simulink model "EV_Regenerative_Braking_Test_FINAL"  (R2021a)
settings: Solver=VariableStepAuto  StartTime=0.0  StopTime=2  RelTol=1e-3
undefined symbols (not defined in the file): Ion, Lithium
libraries: spsBatteryLib x1, pid_lib x1, spsDCMachineLib x1, eePwmGenerator x1, spsTwoQuadrantDCDCConverterLib x1, spsVoltageMeasurementLib x1, spspowerguiLib x1
settings Model: Creator=Adrija  LastModifiedBy=Adrija

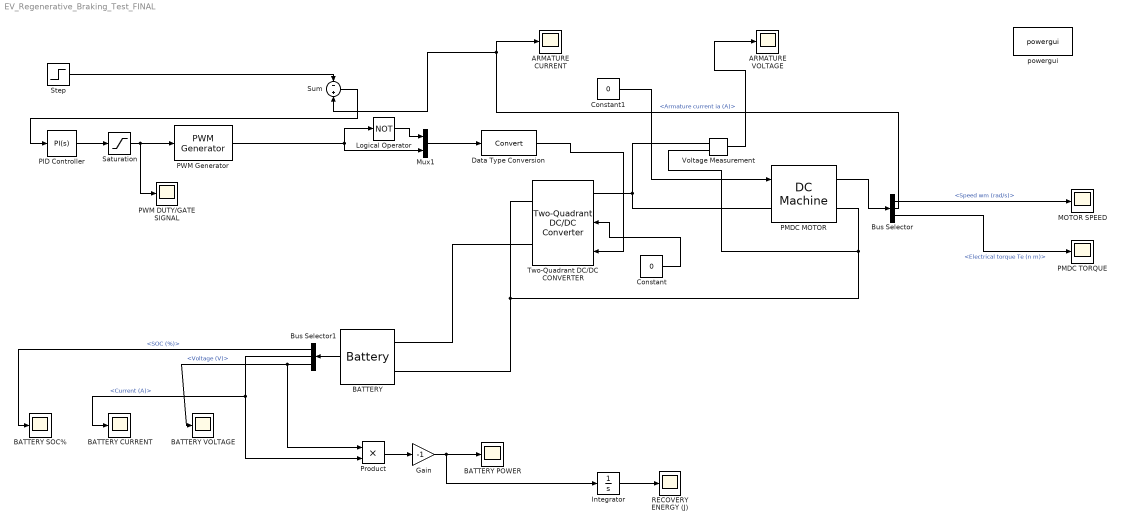
== system EV_Regenerative_Braking_Test_FINAL ==
  ARMATURE CURRENT : Scope
  ARMATURE VOLTAGE : Scope
  BATTERY : spsBatteryLib/Battery  BatType=Lithium-Ion  ShowTempParam=off  ThermalPreset=no  ShowAgeParam=off  NomV=12  NomQ=5.4  SOC=80  Batt_Tr=30  PresetModel=on  MaxQ=5.4  MinV=9  FullV=13.9678  Dis_rate=2.3478  R=0.022222  Normal_OP=4.8835  expZone="[12.9646     0.265304]"  current=[6.5 13 32.5]  Units=Time  Tci=20  NomT=20  T2=-30  MaxQ2=4.8  FullV2=7.1  Normal_OP2=5.655  expZone2="[6.58           1]"  Rca=0.6  ti=2000  Dp=0  Neq0=0  Tsim=1e6  Ta1=25  Qeol=5.4*0.9  Reol=0.013333*1.2  Char_age=[2.3478, 3]  Dis_age=[2.3478, 10]  N1=1500  N2=10500  N3=1000  N4=1400  Ta2=45  N5=950
  BATTERY CURRENT : Scope
  BATTERY POWER : Scope
  BATTERY SOC% : Scope
  BATTERY VOLTAGE : Scope
  Bus Selector : BusSelector  OutputSignals=Speed wm (rad/s),Armature current ia (A),Electrical torque Te (n m)
  Bus Selector1 : BusSelector  OutputSignals=SOC (%),Current (A),Voltage (V)
  Constant : Constant  Value=0
  Constant1 : Constant  Value=0
  Data Type Conversion : DataTypeConversion
  Gain : Gain  Gain=-1
  Integrator : Integrator
  Logical Operator : Logic  Operator=NOT  AllPortsSameDT=off  OutDataTypeStr=boolean
  MOTOR SPEED : Scope
  Mux1 : Mux  Inputs=2
  PID Controller : pid_lib/PID Controller  Controller=PI  Form=Parallel  TimeDomain=Continuous-time  UseExternalTs=off  SampleTime=-1  IntegratorMethod=Forward Euler  FilterMethod=Forward Euler  ControllerParametersSource=internal  P=0.5  I=40  D=0  UseFilter=on  N=100  TunerSelectOption=Transfer Function Based (PID Tuner App)  InitialConditionSource=internal  InitialConditionForIntegrator=0  InitialConditionForFilter=0  DifferentiatorICPrevScaledInput=0  ExternalReset=none  TrackingMode=off  Kt=1  LimitOutput=on  SatLimitsSource=internal  UpperSaturationLimit=1  LowerSaturationLimit=0  LinearizeAsGain=on  AntiWindupMode=back-calculation  Kb=1  RndMeth=Nearest  POutMin=[]  POutMax=[]  IOutMin=[]  IOutMax=[]  DOutMin=[]  DOutMax=[]  NOutMin=[]  NOutMax=[]  SumOutMin=[]  SumOutMax=[]  SaturationOutMin=[]  SaturationOutMax=[]  PParamMin=[]  PParamMax=[]  IParamMin=[]  IParamMax=[]  DParamMin=[]  DParamMax=[]  NParamMin=[]  NParamMax=[]  KbParamMin=[]  KbParamMax=[]  KtParamMin=[]  KtParamMax=[]  KbOutMin=[]  KbOutMax=[]  KtOutMin=[]  KtOutMax=[]  IntegratorOutMin=[]  IntegratorOutMax=[]  FilterOutMin=[]  FilterOutMax=[]  SumI1OutMin=[]  SumI1OutMax=[]  SumI2OutMin=[]  SumI2OutMax=[]  SumI3OutMin=[]  SumI3OutMax=[]  SumI4OutMin=[]  SumI4OutMax=[]  SumDOutMin=[]  SumDOutMax=[]  DifferentiatorOutMin=[]  DifferentiatorOutMax=[]  FilterDiffOutCoefMin=[]  FilterDiffOutCoefMax=[]  ReciprocalOutMin=[]  ReciprocalOutMax=[]  SumDenOutMin=[]  SumDenOutMax=[]  SumNumOutMin=[]  SumNumOutMax=[]  DivideOutMin=[]  DivideOutMax=[]  UdiffTsProdOutMin=[]  UdiffTsProdOutMax=[]  NTsProdOutMin=[]  NTsProdOutMax=[]  UintegralTsProdOutMin=[]  UintegralTsProdOutMax=[]  UngainTsProdOutMin=[]  UngainTsProdOutMax=[]  IntegratorContinuousStateAttributes=''  IntegratorStateMustResolveToSignalObject=off  IntegratorRTWStateStorageClass=Auto  FilterContinuousStateAttributes=''  FilterStateMustResolveToSignalObject=off  FilterRTWStateStorageClass=Auto  ParallelPVariant=InternalParameters  IdealPVariant=Disabled  IVariant=InternalParameters  DVariant=Disabled  IntegratorVariant=Continuous  SatVariant=Enabled  AWVariant=BackCalculation  PCopyVariant=Disabled  TRVariant=Disabled  FdbkBlocksVariant=Forward  IdealPFdbkVariant=Disabled  SatFdbkVariant=Disabled  DerivativeFilterVariant=Disabled  NVariant=Disabled  NCopyVariant=Disabled_SignalSpec  FilterICVariant=Disabled  IntegratorICVariant=InternalICs  ExternalResetVariant=Disabled  TRSumVariant=Passthrough  SumFdbkVariant=Disabled  SumVariant=Sum_PI  TsampFilterVariant=InternalTs  TsampNgainVariant=Passthrough  TsampIntegralVariant=Passthrough  ExternalSaturationOutDataTypeStr=Inherit: Same as second input
  PMDC MOTOR : spsDCMachineLib/DC Machine  PresetModel=No  MechanicalLoad=Torque TL  FieldType=Permanent magnet  ShowDetailedParameters=on  MeasurementBus=off  RLa="[ 0.392  0.012]"  RLf="[ 240  120]"  Laf=1.8  MachineConstant=Torque constant (N.m/A)  Ke=1.8  Kt=0.0597  J=0.01  Bm=0.001  Tf=0  w0=314.16  Ifinit=1  TsPowergui=0  TsBlock=-1
  PMDC TORQUE : Scope
  PWM DUTY/GATE SIGNAL : Scope
  PWM Generator : eePwmGenerator/PWM Generator  CarrCount=Up  Tper=6.6667e-5  Ts=2e-6
  Product : Product
  RECOVERY ENERGY (J) : Scope
  Saturation : Saturate  UpperLimit=1  LowerLimit=0
  Step : Step  Time=0.5  After=-13.4  SampleTime=0
  Sum : Sum  Inputs=-+
  Two-Quadrant DC/DC CONVERTER : spsTwoQuadrantDCDCConverterLib/Two-Quadrant DC//DC Converter  ModelType=Switching devices  Ron=1e-3  Rs=1e6  Cs=inf  Vforward=[0,0]  Ron_Diode=1e-3  Rs_Diode=1e6  Cs_Diode=inf  Vf_Diode=1e-3  Rs_CurrentSource=inf
      settings: SourceProductBaseCode=PS
  Voltage Measurement : spsVoltageMeasurementLib/Voltage Measurement  PhasorSimulation=off  OutputType=Complex  PSBequivalent=0
  powergui : spspowerguiLib/powergui  Priority=1  SimulationMode=Continuous  SampleTime=50e-6  frequency=60  Iterations=50  frequencyindice=0  Pbase=100e6  ErrMax=1e-4  UnitsV=kV  UnitsW=MW  buscounter=0  FunctionMessages=off  echomessages=off  EnableUseOfTLC=off  CurrentSourceSwitches=off  DisableSnubberDevices=off  DisableRonSwitches=off  DisableVfSwitches=off  DisplayEquations=off  AutomaticDiscreteSolvers=off  SolverType=Tustin/Backward Euler (TBE)  Interpol=off  ExternalGateDelay=off  methode=off  Ts=100  x0status=blocks  SPID=on  SwTol=0  HookPort=off  NonlinearTolerance=1e-4  nMaxIteration=100  ContinueOnMaxIteration=off  RestoreLinks=warning  ResistiveCurrentMeasurement=off  Frange=[0:2:500]  Ylog=off  Xlog=on  ShowGrid=off  save=off  variable=ZData  structure=0  ZoomFFT=off  StartTime=0.0  cycles=1  DisplayStyle=1  fundamental=60  FreqAxis=off  MaxFrequency=1000  frequencyindicesteady=1  RmsSteady=1  display=off
  wires:
  PMDC MOTOR/1 -> Bus Selector/1
  Bus Selector/1 -> MOTOR SPEED/1  "<Speed wm (rad/s)>"
  Bus Selector/2 -> Sum/2, ARMATURE CURRENT/1  "<Armature current ia (A)>"
  Bus Selector/3 -> PMDC TORQUE/1  "<Electrical torque Te (n m)>"
  Constant/1 -> Two-Quadrant DC/DC CONVERTER/2
  Constant1/1 -> PMDC MOTOR/1
  Mux1/1 -> Data Type Conversion/1
  BATTERY/1 -> Bus Selector1/1
  Bus Selector1/1 -> BATTERY SOC%/1  "<SOC (%)>"
  Voltage Measurement/1 -> ARMATURE VOLTAGE/1
  Step/1 -> Sum/1
  Sum/1 -> PID Controller/1
  PID Controller/1 -> Saturation/1
  Saturation/1 -> PWM DUTY/GATE SIGNAL/1, PWM Generator/1
  PWM Generator/1 -> Mux1/2, Logical Operator/1
  Logical Operator/1 -> Mux1/1
  Data Type Conversion/1 -> Two-Quadrant DC/DC CONVERTER/1
  Bus Selector1/2 -> Product/2, BATTERY CURRENT/1  "<Current (A)>"
  Bus Selector1/3 -> Product/1, BATTERY VOLTAGE/1  "<Voltage (V)>"
  Product/1 -> Gain/1
  Gain/1 -> Integrator/1, BATTERY POWER/1
  Integrator/1 -> RECOVERY ENERGY (J)/1
  connections:
  Voltage Measurement/LConn1 -- PMDC MOTOR/LConn1 -- Two-Quadrant DC/DC CONVERTER/LConn1
  Two-Quadrant DC/DC CONVERTER/RConn2 -- Voltage Measurement/LConn2 -- PMDC MOTOR/RConn1 -- BATTERY/LConn2
  Two-Quadrant DC/DC CONVERTER/RConn1 -- BATTERY/LConn1
